simulink model "Assignment_3"  (R2020b)
settings: Solver=VariableStepAuto  StartTime=0.0  StopTime=10.0  RelTol=1e-3
values from neighbouring files (symbols this model uses):
  B = 50.0    [Dict_Assignment_3.sldd]
  M = 1000.0    [Dict_Assignment_3.sldd]
settings Model: DataDictionary=Dict_Assignment_3.sldd  Creator=Shantam Garg  LastModifiedBy=Shantam Garg

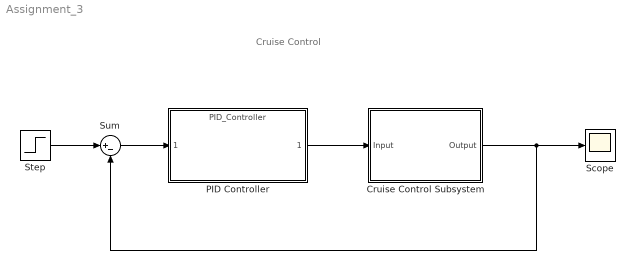
== system Assignment_3 ==
  note: Cruise Control
  Cruise Control Subsystem : Subsystem
  PID Controller : ModelReference  ModelNameDialog=PID_Controller  SimulationMode=Normal  ModelReferenceVersion=1.6
  Scope : Scope
  Step : Step  Time=0  After=u  SampleTime=0
  Sum : Sum  Inputs=|+-
  wires:
  Cruise Control Subsystem/1(Output) -> Scope/1, Sum/2
  Step/1 -> Sum/1
  Sum/1 -> PID Controller/1
  PID Controller/1 -> Cruise Control Subsystem/1(Input)

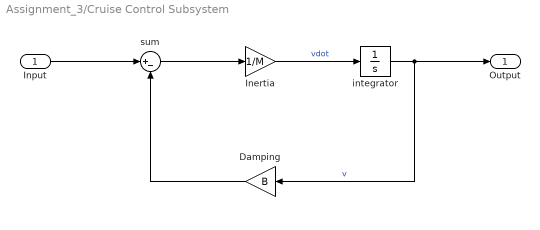
== system Assignment_3/Cruise Control Subsystem ==
  Input : Inport
  Damping : Gain  Gain=B
  Inertia : Gain  Gain=1/M
  integrator : Integrator
  sum : Sum  Inputs=|+-
  Output : Outport
  wires:
  sum/1 -> Inertia/1
  integrator/1 -> Output/1, Damping/1  "v"
  Inertia/1 -> integrator/1  "vdot"
  Damping/1 -> sum/2
  Input/1 -> sum/1
